simulink model "main"  (R2021a)
settings: Solver=VariableStepAuto  StartTime=0.0  StopTime=Torb  RelTol=1e-3
values from neighbouring files (symbols this model uses):
  Ix = Isc(1,1)    [aocs_sim.m]
  Iy = Isc(2,2)    [aocs_sim.m]
  Iz = Isc(3,3)    [aocs_sim.m]
  mu = 3.986e+5    (= 398600)    [aocs_sim.m]
  r0 = [rmag; 0; 0]    [aocs_sim.m]
  v0 = [0; sqrt(mu/rmag); 0]    [aocs_sim.m]
undefined symbols (not defined in the file or in its folder): q0, w0
settings Model: Creator=Laura  LastModifiedBy=Laura

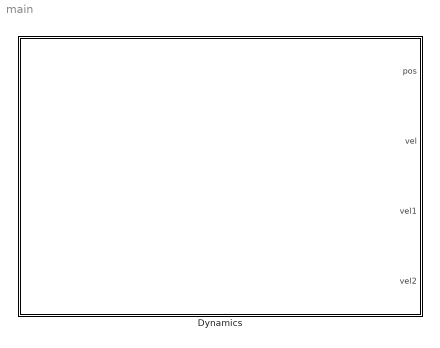
== system main ==
  Dynamics : Subsystem

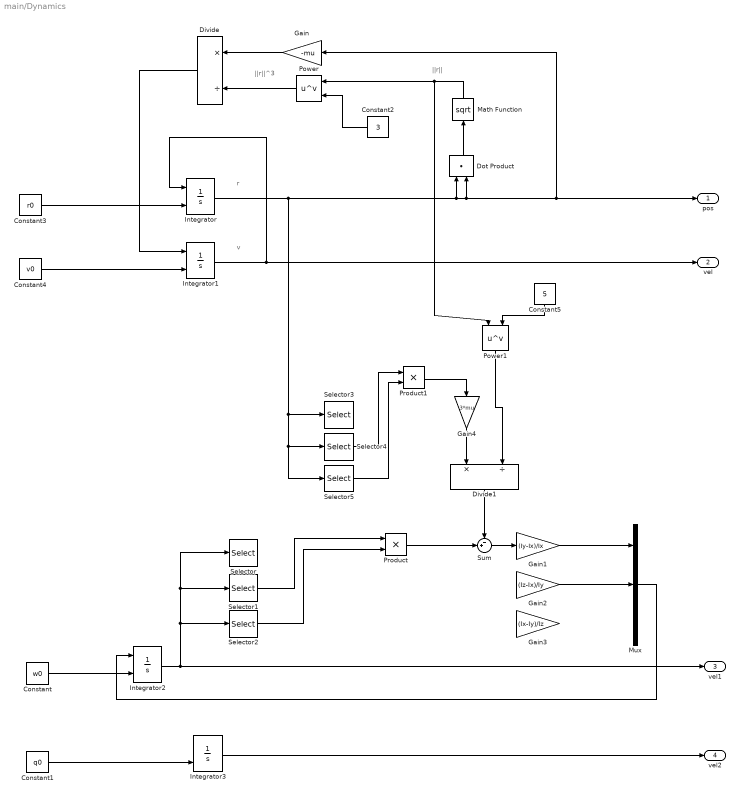
== system main/Dynamics ==
  note: r
  note: v
  note: ||r||^3
  note: ||r||
  Constant : Constant  Value=w0
  Constant1 : Constant  Value=q0
  Constant2 : Constant  Value=3
  Constant3 : Constant  Value=r0
  Constant4 : Constant  Value=v0
  Constant5 : Constant  Value=5
  Divide : Product  Inputs=*/
  Divide1 : Product  Inputs=*/
  Dot Product : DotProduct  InputSameDT=on  OutDataTypeStr=Inherit: Inherit via internal rule
  Gain : Gain  Gain=-mu
  Gain1 : Gain  Gain=(Iy-Ix)/Ix
  Gain2 : Gain  Gain=(Iz-Ix)/Iy
  Gain3 : Gain  Gain=(Ix-Iy)/Iz
  Gain4 : Gain  Gain=3*mu
  Integrator{,1..3} (4 alike) : Integrator  InitialConditionSource=external
  Math Function : Math  Operator=sqrt  SignedPower=on  SaturateOnIntegerOverflow=on
  Mux : Mux  Inputs=3
  Power : Math  Operator=pow  SaturateOnIntegerOverflow=on
  Power1 : Math  Operator=pow  SaturateOnIntegerOverflow=on
  Product : Product
  Product1 : Product
  Selector : Selector  InputPortWidth=3  IndexOptions=Index vector (dialog)  Indices=[1]  OutputSizes=1
  Selector1 : Selector  InputPortWidth=3  IndexOptions=Index vector (dialog)  Indices=[2]  OutputSizes=1
  Selector2 : Selector  InputPortWidth=3  IndexOptions=Index vector (dialog)  Indices=[3]  OutputSizes=1
  Selector3 : Selector  InputPortWidth=3  IndexOptions=Index vector (dialog)  Indices=[1]  OutputSizes=1
  Selector4 : Selector  InputPortWidth=3  IndexOptions=Index vector (dialog)  Indices=[2]  OutputSizes=1
  Selector5 : Selector  InputPortWidth=3  IndexOptions=Index vector (dialog)  Indices=[3]  OutputSizes=1
  Sum : Sum  Inputs=-+|
  pos : Outport
  vel : Outport  Port=2
  vel1 : Outport  Port=3
  vel2 : Outport  Port=4
  wires:
  Math Function/1 -> Power/1, Power1/1
  Constant3/1 -> Integrator/2
  Constant2/1 -> Power/2
  Integrator1/1 -> vel/1, Integrator/1
  Integrator/1 -> Dot Product/1, Dot Product/2, pos/1, Gain/1, Selector3/1, Selector4/1, Selector5/1
  Dot Product/1 -> Math Function/1
  Gain/1 -> Divide/1
  Divide/1 -> Integrator1/1
  Constant4/1 -> Integrator1/2
  Power/1 -> Divide/2
  Constant1/1 -> Integrator3/2
  Constant/1 -> Integrator2/2
  Integrator2/1 -> vel1/1, Selector2/1, Selector1/1, Selector/1
  Integrator3/1 -> vel2/1
  Mux/1 -> Integrator2/1
  Gain1/1 -> Mux/1
  Gain2/1 -> Mux/2
  Product/1 -> Sum/2
  Sum/1 -> Gain1/1
  Selector2/1 -> Product/2
  Selector1/1 -> Product/1
  Constant5/1 -> Power1/2
  Divide1/1 -> Sum/1
  Product1/1 -> Gain4/1
  Gain4/1 -> Divide1/1
  Power1/1 -> Divide1/2
  Selector4/1 -> Product1/1
  Selector5/1 -> Product1/2
